simulink model "regulacjapred"  (R2013a)
settings: Solver=ode45  StartTime=0.0  StopTime=5  RelTol=1e-3
values from neighbouring files (symbols this model uses):
  B = T    (= 0.0283333333333)    [pred.m]
  J = 0.089    [pred.m]
  ksi = 220*0.175*sqrt(2)    [pred.m]
  kt = 0.04    [pred.m]
  kw = J*kz/(2*B*kt*ksi*0.175)    [pred.m]
  kz = 1/Rs    (= 3.33333333333)    [pred.m]
  Tm = 0.005    [pred.m]
  tw = 4*B    (= 0.113333333333)    [pred.m]
libraries: simulink x1, powerlib x1
settings Model: Creator=Martial NGAHA  LastModifiedBy=Martial NGAHA

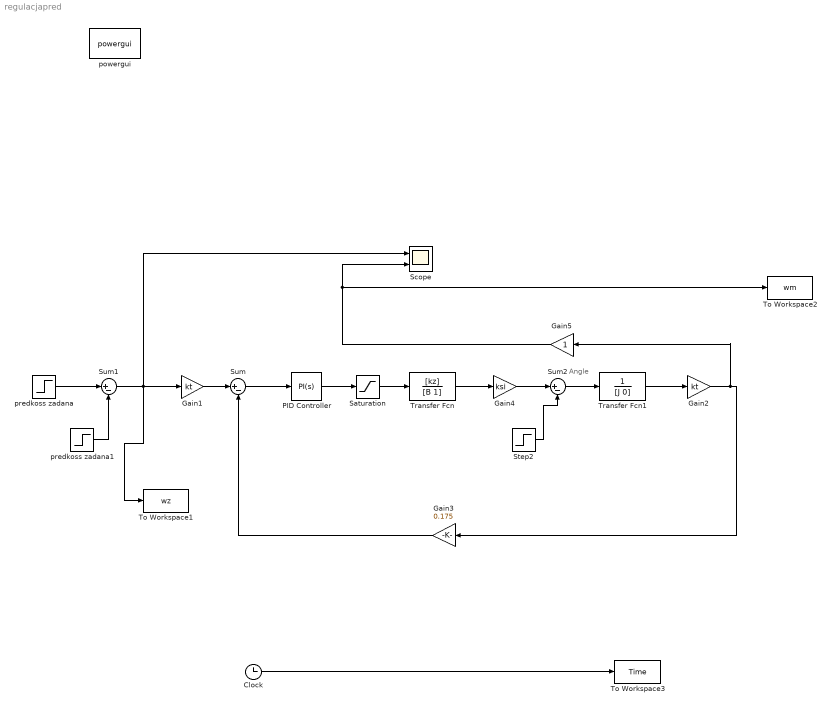
== system regulacjapred ==
  note: Angle
  Clock : Clock
  Gain1 : Gain  Gain=kt  SampleTime=0
  Gain2 : Gain  Gain=kt  SampleTime=0
  Gain3 : Gain  Gain=0.175  SampleTime=0
  Gain4 : Gain  Gain=ksi  SampleTime=0
  Gain5 : Gain  SampleTime=0
  PID Controller : simulink/Continuous/PID Controller  Controller=PI  TimeDomain=Continuous-time  SampleTime=1  IntegratorMethod=Forward Euler  FilterMethod=Forward Euler  Form=Parallel  P=kw  I=kw/tw  D=0  N=100  InitialConditionSource=internal  InitialConditionForIntegrator=0  InitialConditionForFilter=0  ExternalReset=none  LimitOutput=off  UpperSaturationLimit=inf  LowerSaturationLimit=-inf  LinearizeAsGain=on  AntiWindupMode=none  Kb=1  TrackingMode=off  Kt=1  PParamMin=[]  PParamMax=[]  IParamMin=[]  IParamMax=[]  DParamMin=[]  DParamMax=[]  NParamMin=[]  NParamMax=[]  KbParamMin=[]  KbParamMax=[]  KtParamMin=[]  KtParamMax=[]  POutMin=[]  POutMax=[]  IOutMin=[]  IOutMax=[]  DOutMin=[]  DOutMax=[]  NOutMin=[]  NOutMax=[]  KbOutMin=[]  KbOutMax=[]  KtOutMin=[]  KtOutMax=[]  IntegratorOutMin=[]  IntegratorOutMax=[]  FilterOutMin=[]  FilterOutMax=[]  SumOutMin=[]  SumOutMax=[]  SumI1OutMin=[]  SumI1OutMax=[]  SumI2OutMin=[]  SumI2OutMax=[]  SumI3OutMin=[]  SumI3OutMax=[]  SumDOutMin=[]  SumDOutMax=[]  SaturationOutMin=[]  SaturationOutMax=[]  IntegratorContinuousStateAttributes=''  IntegratorStateMustResolveToSignalObject=off  IntegratorRTWStateStorageClass=Auto  FilterContinuousStateAttributes=''  FilterStateMustResolveToSignalObject=off  FilterRTWStateStorageClass=Auto
  Saturation : Saturate  UpperLimit=120  LowerLimit=-120  SampleTime=0
  Scope : Scope  NumInputPorts=2
      settings: YMin=-5~-5  YMax=5~5
  Step2 : Step  Time=2  After=Tm  SampleTime=0
  Sum : Sum  Inputs=|+-  SampleTime=0
  Sum1 : Sum  Inputs=|+-
  Sum2 : Sum  Inputs=|+-
  To Workspace1 : ToWorkspace  VariableName=wz  SaveFormat=Structure With Time
  To Workspace2 : ToWorkspace  VariableName=wm  SaveFormat=Structure With Time
  To Workspace3 : ToWorkspace  VariableName=Time  SaveFormat=Structure With Time
  Transfer Fcn : TransferFcn  Numerator=[kz]  Denominator=[B 1]
  Transfer Fcn1 : TransferFcn  Denominator=[J 0]
  powergui : powerlib/powergui  Priority=1  SimulationMode=Discrete  SolverType=Tustin  SampleTime=1e-6  frequency=60  SPID=off  DisableSnubberDevices=off  DisableRonSwitches=off  DisableVfSwitches=off  SwTol=0  Interpol=off  DisplayEquations=off  frequencyindice=60  Pbase=100e6  ErrMax=1e-4  Iterations=50  UnitsV=kV  UnitsW=MW  FunctionMessages=off  echomessages=off  HookPort=off  EnableUseOfTLC=off  x0status=blocks  RestoreLinks=warning  ResistiveCurrentMeasurement=off  Frange=[0:2:500]  Ylog=off  Xlog=on  ShowGrid=off  save=off  variable=ZData  ZoomFFT=off  StartTime=0.0  cycles=1  DisplayStyle=1  fundamental=60  FreqAxis=off  MaxFrequency=1000  frequencyindicesteady=1  RmsSteady=1  display=off  Ts=0  methode=off
  predkoss zadana : Step  Time=0  After=3000
  predkoss zadana1 : Step  After=6000
  wires:
  Step2/1 -> Sum2/2
  Gain4/1 -> Sum2/1
  Transfer Fcn/1 -> Gain4/1
  Gain3/1 -> Sum/2
  Sum/1 -> PID Controller/1
  Sum2/1 -> Transfer Fcn1/1
  PID Controller/1 -> Saturation/1
  Clock/1 -> To Workspace3/1
  Transfer Fcn1/1 -> Gain2/1
  Saturation/1 -> Transfer Fcn/1
  Gain1/1 -> Sum/1
  Gain2/1 -> Gain5/1, Gain3/1
  Gain5/1 -> To Workspace2/1, Scope/2
  predkoss zadana/1 -> Sum1/1
  predkoss zadana1/1 -> Sum1/2
  Sum1/1 -> To Workspace1/1, Scope/1, Gain1/1
